simulink model "power_PVarray_250kW_modified_R2020a"  (R2020a)
settings: Solver=VariableStepAuto  StartTime=0.0  StopTime=10  RelTol=1e-3
PreLoadFcn:
  | power_PVarray_250kW_param;
InitFcn:
  | power_PVarray_250kW_param;
undefined symbols (not defined in the file): Clink, D1, Delta, Fc, Fnom, Increment_MPPT, Ion, Ki_Ireg, Ki_VDCreg, Kp_Ireg, Kp_VDCreg, LimitL_Ireg, LimitL_VDCreg, Limits_MPPT, LimitU_Ireg, LimitU_VDCreg, Lithium, Pnom, Pnom_xfo, RL, RLff, sigbuilder_block, Ts_Control, Ts_Power, Vf, Vfd, Vnom_dc, Vnom_prim, Vnom_sec
libraries: powerlib x24, powerlib_meascontrol x10, simulink x4, electricdrivelib x1, re_lib x1
(part 2 of 2)

== matlab function power_PVarray_250kW_modified_R2020a/Inverter Control/MPPT Controller using Perturbe & Observe technique  ==
  settings: updateMethod=DISCRETE  sampleTime=Ts_Control
  data: Param input; Enabled input; V input; I input; D output
function D  = PandO(Param, Enabled, V, I)

% MPPT controller based on the Perturb & Observe algorithm.

% D output = Reference for DC link voltage (Vdc_ref) 
%
% Enabled input = 1 to enable the MPPT controller
% V input = PV array terminal voltage (V)
% I input = PV array current (A)
%
% Param input:
Dinit = Param(1);  %Initial value for Vdc_ref
Dmax = Param(2);   %Maximum value for Vdc_ref
Dmin = Param(3);   %Minimum value for Vdc_ref
deltaD = Param(4); %Increment value used to increase/decrease Vdc_ref
%  

persistent Vold Pold Dold;

dataType = 'double';

if isempty(Vold)
    Vold=0;
    Pold=0;
    Dold=Dinit;
end
P= V*I;
dV= V - Vold;
dP= P - Pold;

if dP ~= 0 & Enabled ~=0
    if dP < 0
        if dV < 0
            D = Dold + deltaD;
        else
            D = Dold - deltaD;
        end
    else
        if dV < 0
            D = Dold - deltaD;
        else
            D = Dold + deltaD;
        end    
    end
else D=Dold;
end

if D >= Dmax | D<= Dmin
    D=Dold;
end

Dold=D;
Vold=V;
Pold=P;
